simulink model "generate_joint_velocity_motion"  (R2023a)
settings: Solver=FixedStepDiscrete  StartTime=0.0  StopTime=inf  FixedStep=0.001  RelTol=1e-3  EnableMultiTasking=on
PreLoadFcn:
  | frs = FrankaRobotSettings;
undefined symbols (not defined in the file): DiscIntNeverNeededParam
libraries: franka_simulink_library x3
settings Model: SimulationMode=external  ExtModeTrigDuration=10000  Creator=vasi_ko  LastModifiedBy=kvasios
settings SolverCC: AlgebraicLoopSolver=TrustRegion
settings DataIOCC: LimitDataPoints=on  SaveFormat=Array  ReturnWorkspaceOutputs=off
settings OptimizationCC: EnhancedBackFolding=on  PassReuseOutputArgsThreshold=0  MaxStackSize=64  OptimizeBlockOrder=speed  DifferentSizesBufferReuse=on  OptimizationCustomize=off
settings DebuggingCC: SolverPrmCheckMsg=warning  ParameterTunabilityLossMsg=error  UnconnectedInputMsg=warning  UnconnectedOutputMsg=warning  UnconnectedLineMsg=warning  SFUnexpectedBacktrackingDiag=warning  SFNoUnconditionalDefaultTransitionDiag=warning  SFExecutionAtInitializationDiag=none  ArithmeticOperatorsInVariantConditions=warning
settings ModelReferenceCC: EnableRefExpFcnMdlSchedulingChecks=on  PropagateSignalLabelsOutOfModel=off
settings SFSimCC: SimUseLocalCustomCode=off  MATLABDynamicMemAlloc=off  CustomCodeUndefinedFunction=UseInterfaceOnly  SimTargetLang=C++
settings RTWCC: RTWVerbose=off  RTWUseLocalCustomCode=off  BuildConfiguration=Faster Runs  TargetLang=C++  DLArmComputeVersion=19.05
settings CodeAppCC: ForceParamTrailComments=on  OperatorAnnotations=on
settings ConfigComp: CovMetricSettings=dw  CovSaveCumulativeToWorkspaceVar=on  CovSaveSingleToWorkspaceVar=on  CovExternalEMLEnable=off  CovSFcnEnable=off

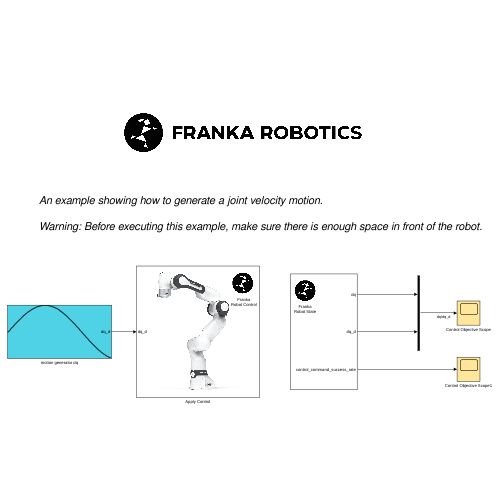
[thumbnail: Simulink's stored preview of the top-level diagram]
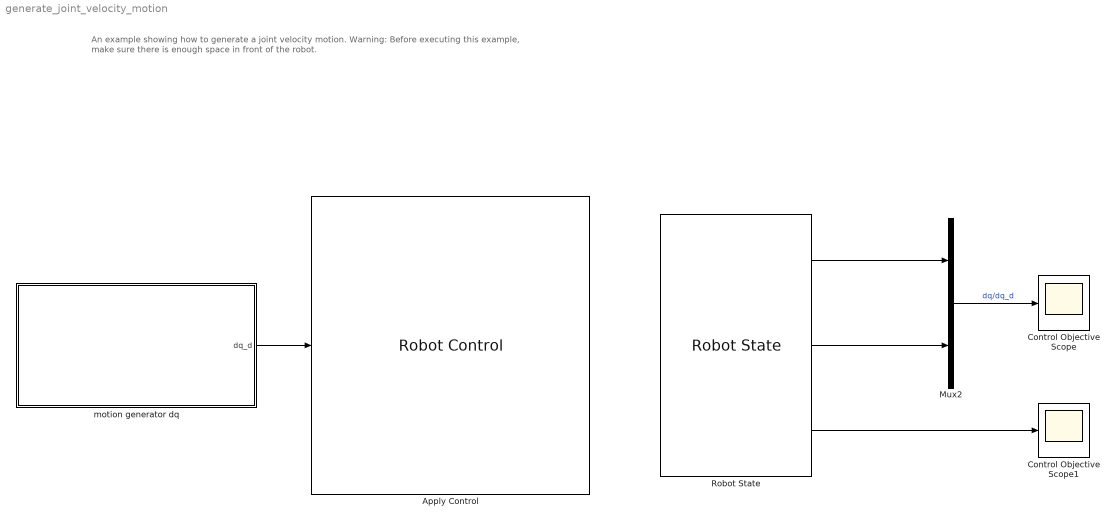
== system generate_joint_velocity_motion ==
  note: An example showing how to generate a joint velocity motion.
      |
      | Warning: Before executing this example, make sure there is enough space in front of the robot.
  Apply Control : franka_simulink_library/Robot Control  robot_ip=frs.robot_ip  gripper_selection=None  control_mode=Joint Velocities - Internal Controller Mode  controller_choice=Joint Impedance Controller  joint_impedance=frs.joint_impedance_stiffness  cartesian_impedance=[3000, 3000, 3000, 300, 300, 300]  rate_limiter=on  cuttoff_frequency=frs.cutoff_frequency  elbow_control=off  collision_thresholds=frs.collision_thresholds.getAs1DArray  load_inertia=frs.load_inertia.getAs1DArray  NE_T_EE=frs.NE_T_EE(:)  EE_T_K=frs.EE_T_K(:)  init_joint_configuration_req=on  init_joint_configuration=frs.home_configuration
      settings: SourceProductName=Franka Robotics Simulink Support Package
  Control Objective Scope : Scope
  Control Objective Scope1 : Scope
  Mux2 : Mux  Inputs=2
  Robot State : franka_simulink_library/Robot State  robot_ip=frs.robot_ip  signals_requested='dq dq_d control_command_success_rate'
      settings: SourceProductName=Franka Robotics Simulink Support Package
  motion generator dq : Subsystem
      mask Display:
      | pos = get_param(gcb, 'Position');
      | width = pos(3) - pos(1);
      | x = [0:width];
      | y = sin(x/180*pi);
      | % Parameters 'm' and 'b' must be defined in 'Parameters & Dialog' pane.
      | plot(x,y );
      | 
      | port_label('output',1,'dq_d');
  wires:
  Robot State/1 -> Mux2/1
  Robot State/2 -> Mux2/2
  Mux2/1 -> Control Objective Scope/1  "dq/dq_d"
  motion generator dq/1(dq_d) -> Apply Control/1
  Robot State/3 -> Control Objective Scope1/1

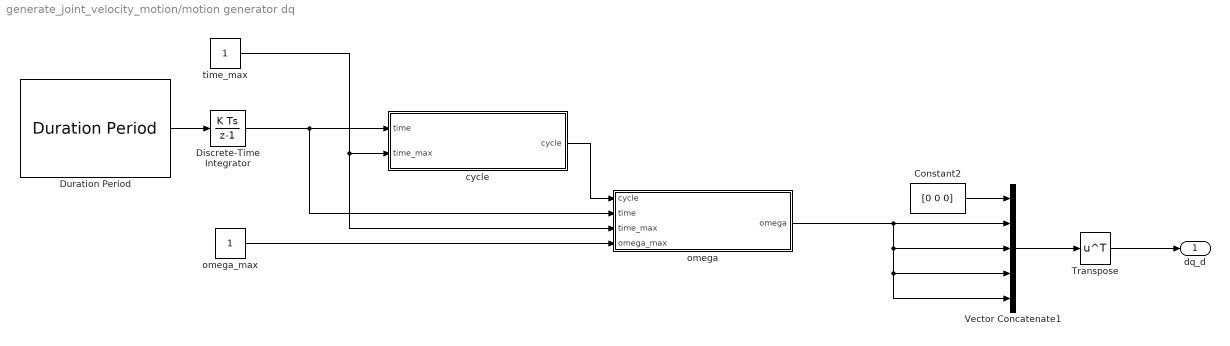
== system generate_joint_velocity_motion/motion generator dq ==
  Constant2 : Constant  Value=[0 0 0]  VectorParams1D=off
  Discrete-Time Integrator : DiscreteIntegrator  gainval=1000  SampleTime=0.001  ICPrevOutput=DiscIntNeverNeededParam  ICPrevScaledInput=DiscIntNeverNeededParam
  Duration Period : franka_simulink_library/Duration Period  robot_ip=frs.robot_ip
      settings: SourceProductName=Franka Robotics Simulink Support Package
  Transpose : Math  Operator=transpose
  Vector Concatenate1 : Concatenate  NumInputs=5
  cycle : Subsystem
  omega : Subsystem
  omega_max : Constant  VectorParams1D=off
  time_max : Constant  VectorParams1D=off
  dq_d : Outport  VectorParamsAs1DForOutWhenUnconnected=off
  wires:
  Constant2/1 -> Vector Concatenate1/1
  Duration Period/1 -> Discrete-Time Integrator/1
  Vector Concatenate1/1 -> Transpose/1
  omega/1(omega) -> Vector Concatenate1/5, Vector Concatenate1/4, Vector Concatenate1/3, Vector Concatenate1/2
  time_max/1 -> omega/3(time_max), cycle/2(time_max)
  cycle/1(cycle) -> omega/1(cycle)
  omega_max/1 -> omega/4(omega_max)
  Discrete-Time Integrator/1 -> cycle/1(time), omega/2(time)
  Transpose/1 -> dq_d/1

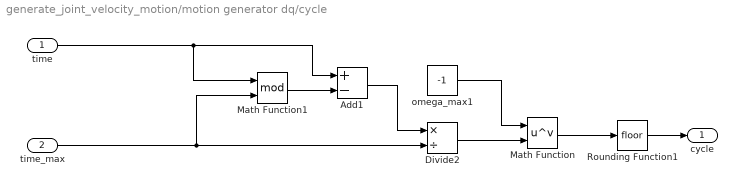
== system generate_joint_velocity_motion/motion generator dq/cycle ==
  time : Inport
  time_max : Inport  Port=2
  Add1 : Sum  Inputs=+-
  Divide2 : Product  Inputs=*/
  Math Function : Math  Operator=pow  SignedPower=on
  Math Function1 : Math  Operator=mod  SignedPower=on
  Rounding Function1 : Rounding
  omega_max1 : Constant  Value=-1  VectorParams1D=off
  cycle : Outport  InitialOutput=[0 0 0 0 0 0 0]  VectorParamsAs1DForOutWhenUnconnected=off
  wires:
  Divide2/1 -> Math Function/2
  Math Function1/1 -> Add1/2
  time/1 -> Add1/1, Math Function1/1
  time_max/1 -> Math Function1/2, Divide2/2
  Rounding Function1/1 -> cycle/1
  Math Function/1 -> Rounding Function1/1
  omega_max1/1 -> Math Function/1
  Add1/1 -> Divide2/1

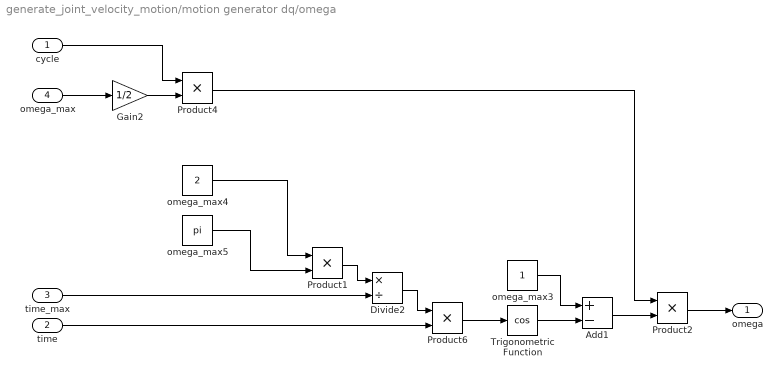
== system generate_joint_velocity_motion/motion generator dq/omega ==
  cycle : Inport
  time : Inport  Port=2
  time_max : Inport  Port=3
  omega_max : Inport  Port=4
  Add1 : Sum  Inputs=+-
  Divide2 : Product  Inputs=*/
  Gain2 : Gain  Gain=1/2
  Product{1..2,4,6} (4 alike) : Product
  Trigonometric Function : Trigonometry  Operator=cos
  omega_max3 : Constant  VectorParams1D=off
  omega_max4 : Constant  Value=2  VectorParams1D=off
  omega_max5 : Constant  Value=pi  VectorParams1D=off
  omega : Outport  InitialOutput=[0 0 0 0 0 0 0]  VectorParamsAs1DForOutWhenUnconnected=off
  wires:
  cycle/1 -> Product4/1
  omega_max/1 -> Gain2/1
  Product4/1 -> Product2/1
  Gain2/1 -> Product4/2
  omega_max3/1 -> Add1/1
  omega_max5/1 -> Product1/2
  omega_max4/1 -> Product1/1
  Divide2/1 -> Product6/1
  Product1/1 -> Divide2/1
  Product6/1 -> Trigonometric Function/1
  Trigonometric Function/1 -> Add1/2
  time_max/1 -> Divide2/2
  time/1 -> Product6/2
  Add1/1 -> Product2/2
  Product2/1 -> omega/1
